simulink model "bungee"  (R2014b)
settings: Solver=ode45  StartTime=0.0  StopTime=30.0  RelTol=1e-3
settings Model: Creator=csimon  LastModifiedBy=csimon

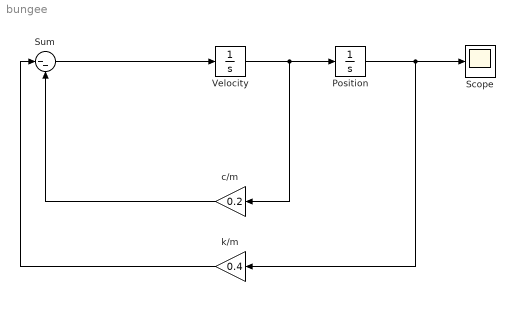
== system bungee ==
  Position : Integrator  InitialCondition=1
  Scope : Scope
  Sum : Sum  Inputs=|--
  Velocity : Integrator  InitialCondition=1
  c/m : Gain  Gain=0.2
  k/m : Gain  Gain=0.4
  wires:
  c/m/1 -> Sum/2
  k/m/1 -> Sum/1
  Sum/1 -> Velocity/1
  Velocity/1 -> c/m/1, Position/1
  Position/1 -> k/m/1, Scope/1
